simulink subsystem "state_machine"  (R2019b)
settings: Solver=VariableStepAuto  StartTime=0.0  StopTime=10.0  RelTol=1e-3
settings Model: Creator=andrea  LastModifiedBy=andrea

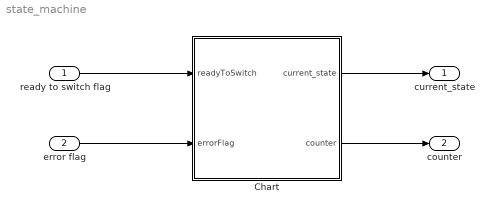
== system state_machine ==
  ready to switch flag : Inport
  error flag : Inport  Port=2
  Chart : Stateflow chart  BlockKeywords=__PRM__SERIALIZED__DATA__:Stateflow Chart,Stateflow Diagram  TreatAsAtomicUnit=on
  current_state : Outport
  counter : Outport  Port=2
  wires:
  ready to switch flag/1 -> Chart/1(readyToSwitch)
  error flag/1 -> Chart/2(errorFlag)
  Chart/1(current_state) -> current_state/1
  Chart/2(counter) -> counter/1

== stateflow chart state_machine/Chart ==
  state inizializzazione
    current_state = 0
  state ispezione
    state pre_ispezione
      counter = 1
    state arco
    state verticale
    (default) -> pre_ispezione
    pre_ispezione -> verticale
    verticale -> arco [order 1] : [readyToSwitch]
    arco -> verticale : [readyToSwitch]{counter = counter + 1}
  state errore
    current_state = 500
  state fine
    current_state = 999
  verticale -> fine [order 2] : [counter == 10 && readyToSwitch]
  (default) -> inizializzazione
  inizializzazione -> ispezione [order 1] : [readyToSwitch]
  ispezione -> errore : [errorFlag]
  inizializzazione -> errore [order 2] : [errorFlag]
  fine -> errore : [errorFlag]
  data: readyToSwitch input; errorFlag input; current_state output; counter output; type constant double
